simulink model "ComputerPilot"  (R2023b)
settings: Solver=FixedStepAuto  StartTime=0.0  StopTime=inf  FixedStep=sample_time  RelTol=1e-3
InitFcn:
  | load("drone_buses.mat");
model workspace (MAT data in the model file):
  SL_ROS_VariableLengthArrays_MaxSizes.CommonInfo.ArrayTruncateAction = 'EmitWarning'
  SL_ROS_VariableLengthArrays_MaxSizes.MsgTypeMap = containers.Map
  SL_ROS_VariableLengthArrays_MaxSizes.MsgTypeMap.serialization.keys = {'sensor_msgs/Image'}
  SL_ROS_VariableLengthArrays_MaxSizes.MsgTypeMap.serialization.values{1}(1).PropertyName = 'data'
  SL_ROS_VariableLengthArrays_MaxSizes.MsgTypeMap.serialization.values{1}(1).DataType = 'uint8'
  SL_ROS_VariableLengthArrays_MaxSizes.MsgTypeMap.serialization.values{1}(1).MaxLength = 921600
  SL_ROS_VariableLengthArrays_MaxSizes.MsgTypeMap.serialization.values{1}(2).PropertyName = 'encoding'
  SL_ROS_VariableLengthArrays_MaxSizes.MsgTypeMap.serialization.values{1}(2).DataType = 'uint8'
  SL_ROS_VariableLengthArrays_MaxSizes.MsgTypeMap.serialization.values{1}(2).MaxLength = 128
  SL_ROS_VariableLengthArrays_MaxSizes.MsgTypeMap.serialization.uniformity = 0
  SL_ROS_VariableLengthArrays_MaxSizes.MsgTypeMap.serialization.keyType = 'char'
  SL_ROS_VariableLengthArrays_MaxSizes.MsgTypeMap.serialization.valueType = 'any'
  sample_time = 0.1
undefined symbols (not defined in the file): duration, vel
libraries: ros2lib x5, visionsinks x1
settings Model: Creator=rcasado  LastModifiedBy=Rafa
settings SolverCC: AlgebraicLoopSolver=TrustRegion
settings DataIOCC: ReturnWorkspaceOutputs=off
settings OptimizationCC: EnhancedBackFolding=on  PassReuseOutputArgsAs=Individual arguments  ZeroExternalMemoryAtStartup=off  ZeroInternalMemoryAtStartup=off  MaxStackSize=64  OptimizeBlockOrder=speed  DifferentSizesBufferReuse=on  OptimizationCustomize=off  EfficientTunableParamExpr=on
settings DebuggingCC: ParameterTunabilityLossMsg=error  UnconnectedInputMsg=warning  UnconnectedOutputMsg=warning  UnconnectedLineMsg=warning  BusObjectLabelMismatch=none  PregeneratedLibrarySubsystemCodeDiagnostic=none  ArithmeticOperatorsInVariantConditions=warning
settings HardwareCC: ProdBitPerPointer=32  ProdBitPerSizeT=32  ProdBitPerPtrDiffT=32  ProdLargestAtomicFloat=None  ProdIntDivRoundTo=Undefined  ProdEndianess=Unspecified  ProdWordSize=32  ProdHWDeviceType=Generic->Unspecified (assume 32-bit Generic)
settings ModelReferenceCC: EnableRefExpFcnMdlSchedulingChecks=on
settings SFSimCC: SimUseLocalCustomCode=off  CustomCodeUndefinedFunction=UseInterfaceOnly  SimTargetLang=C++
settings RTWCC: Description=Embedded Coder  SystemTargetFile=ert.tlc  HardwareBoard=Robot Operating System (ROS)  TLCOptions="-aInlineSetEventsForThisBaseRateFcn=TLC_FALSE -aSuppressMultiTaskScheduler=TLC_FALSE  -aRateBasedStepFcn=0"  GenCodeOnly=on  TemplateMakefile=ert_default_tmf  GenerateReport=on  RTWUseLocalCustomCode=off  Toolchain=Catkin  IncludeHyperlinkInReport=on  LaunchReport=on  TargetLang=C++  GenerateTraceInfo=on  GenerateTraceReport=on  GenerateTraceReportSl=on  GenerateTraceReportSf=on  GenerateTraceReportEml=on  DLArmComputeVersion=19.05
settings CodeAppCC: ForceParamTrailComments=on  IgnoreCustomStorageClasses=off  OperatorAnnotations=on  SimulinkDataObjDesc=on  SFDataObjDesc=on  InsertBlockDesc=on

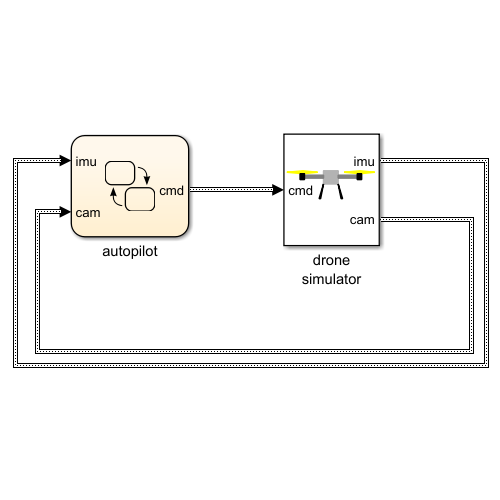
[thumbnail: Simulink's stored preview of the top-level diagram]
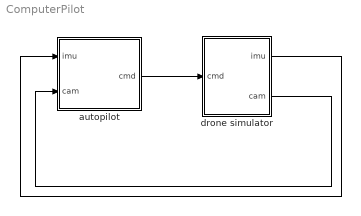
== system ComputerPilot ==
  autopilot : Stateflow chart  TreatAsAtomicUnit=on
  drone simulator : Subsystem
      mask Display:
      | patch([50 -50 -50 50], [40 40 -60 -60], [1 1 1])
      | 
      | patch([8 -8 -8 8], [6 6 -6 -6], [0.7 0.7 0.7])
      | 
      | patch([ 8  8  28  28], [2 0 0 2], [0.5 0.5 0.5])
      | patch([-8 -8 -28 -28], [2 0 0 2], [0.5 0.5 0.5])
      | 
      | patch([ 30  46  30  14], [6 5 4 5], [1 1 0])
      | patch([-30 -46 -30 -14], [6 5 4 5], [1 1 0])
      | 
      | patch([ 28  28  32  32], [4 -2 -2 4], [0 0 0])
      | patch([-28 -28 -32 -32], [4 -2 -2 4], [0 0 0])
      | 
      | patch([ 8  12  11  7], [-6 -18 -18 -6], [0 0 0])
      | patch([-8 -12 -11 -7], [-6 -18 -18 -6], [0 0 0])
  wires:
  drone simulator/1(imu) -> autopilot/1(imu)
  autopilot/1(cmd) -> drone simulator/1(cmd)
  drone simulator/2(cam) -> autopilot/2(cam)

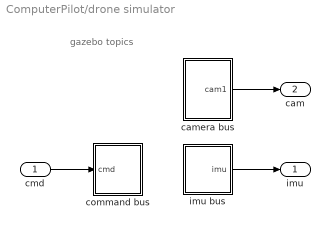
== system ComputerPilot/drone simulator ==
  note: gazebo
      | topics
  cmd : Inport
  camera bus : Subsystem
  command bus : Subsystem
  imu bus : Subsystem
  imu : Outport  VectorParamsAs1DForOutWhenUnconnected=off
  cam : Outport  Port=2  VectorParamsAs1DForOutWhenUnconnected=off
  wires:
  imu bus/1(imu) -> imu/1
  cmd/1 -> command bus/1(cmd)
  camera bus/1(cam1) -> cam/1

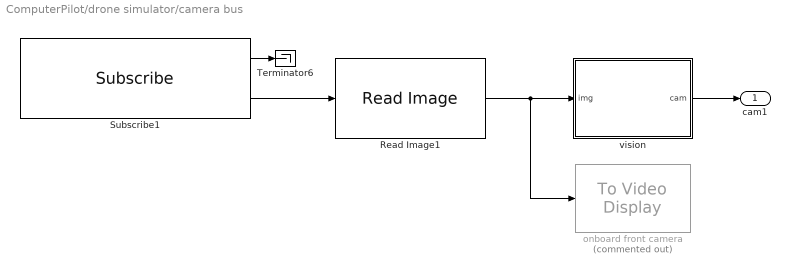
== system ComputerPilot/drone simulator/camera bus ==
  Read Image1 : ros2lib/Read Image  MaximumImageSize=[240, 320]  ImageEncoding=rgb8  ShowAlphaOutput=off  ShowErrorCodeOutput=off  VariableSizeOutputs=off
  Subscribe1 : ros2lib/Subscribe  topicSource=Select from ROS network  topic=/NavSim/abejorro/onboard_cam/image_raw  messageType=sensor_msgs/Image  sampleTime=0.1  QOSHistory=Keep last  QOSDepth=1  QOSReliability=Reliable  QOSDurability=Volatile
  Terminator6 : Terminator
  onboard front camera : visionsinks/To Video Display  Commented=on  windowSizeMode=Normal  openAtMdlStart=on  fullScreen=off  videoWindowX=536805376  videoWindowY=536805376  saveWindowSize=off  videoWindowWidth=479  videoWindowHeight=321  inputColorFormat=RGB  inputType=Obsolete  imagePorts=One multidimensional signal  OutputDevice=On-screen video monitor  dataOrg=Column-major  isWindowOpen=off
  vision : MATLAB Function  TreatAsAtomicUnit=on
  cam1 : Outport  VectorParamsAs1DForOutWhenUnconnected=off
  wires:
  Subscribe1/2 -> Read Image1/1
  vision/1(cam) -> cam1/1
  Subscribe1/1 -> Terminator6/1
  Read Image1/1 -> vision/1(img), onboard front camera/1

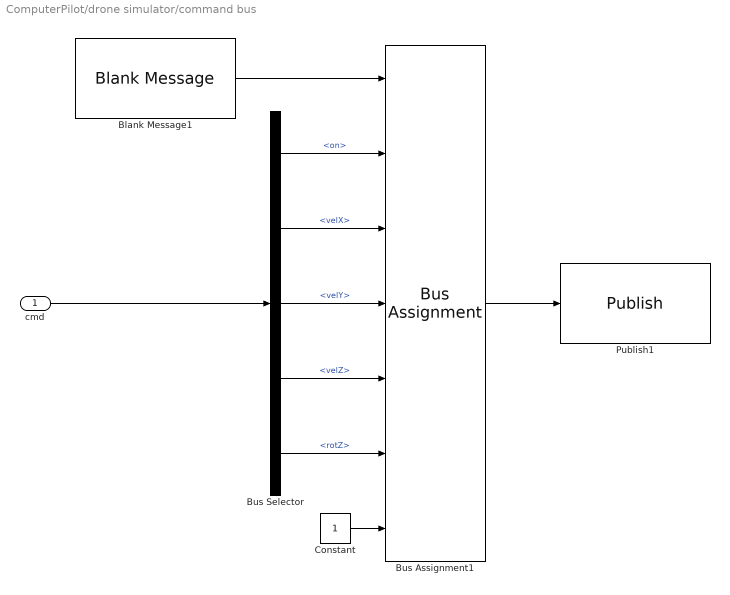
== system ComputerPilot/drone simulator/command bus ==
  cmd : Inport
  Blank Message1 : ros2lib/Blank Message  messageClass=Message  entityType=navsim_msgs/RemoteCommand  messageType=navsim_msgs/RemoteCommand  SampleTime=sample_time
  Bus Assignment1 : BusAssignment  AssignedSignals=on,vel.linear.x,vel.linear.y,vel.linear.z,vel.angular.z,duration.sec
  Bus Selector : BusSelector  OutputSignals=on,velX,velY,velZ,rotZ
  Constant : Constant  OutDataTypeStr=int32
  Publish1 : ros2lib/Publish  topicSource=Select from ROS network  topic=/NavSim/abejorro/RemoteCommand  messageType=navsim_msgs/RemoteCommand  QOSHistory=Keep last  QOSDepth=1  QOSReliability=Reliable  QOSDurability=Volatile
  wires:
  cmd/1 -> Bus Selector/1
  Bus Selector/4 -> Bus Assignment1/5  "<velZ>"
  Bus Selector/3 -> Bus Assignment1/4  "<velY>"
  Bus Selector/2 -> Bus Assignment1/3  "<velX>"
  Bus Selector/1 -> Bus Assignment1/2  "<on>"
  Bus Selector/5 -> Bus Assignment1/6  "<rotZ>"
  Blank Message1/1 -> Bus Assignment1/1
  Bus Assignment1/1 -> Publish1/1
  Constant/1 -> Bus Assignment1/7

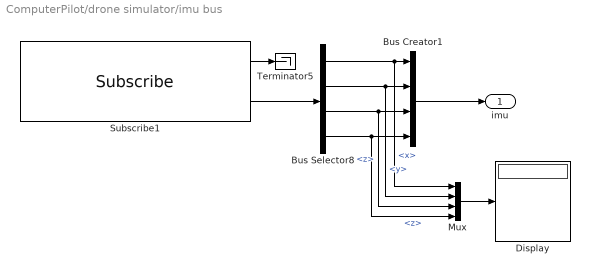
== system ComputerPilot/drone simulator/imu bus ==
  Bus Creator1 : BusCreator  Inputs=4  OutDataTypeStr=Bus: bus_IMU  NonVirtualBus=on
      settings: InheritFromInputs=off
  Bus Selector8 : BusSelector  DialogController=Simulink.DDGSource_BusSelector  OutputSignals=pose.position.x,pose.position.y,pose.position.z,pose.orientation.z
  Display : Display
  Mux : Mux
  Subscribe1 : ros2lib/Subscribe  topicSource=Select from ROS network  topic=/NavSim/abejorro/Telemetry  messageType=navsim_msgs/Telemetry  sampleTime=0.1  QOSHistory=Keep last  QOSDepth=1  QOSReliability=Reliable  QOSDurability=Volatile
  Terminator5 : Terminator
  imu : Outport  VectorParamsAs1DForOutWhenUnconnected=off
  wires:
  Subscribe1/1 -> Terminator5/1
  Bus Selector8/4 -> Mux/4, Bus Creator1/4  "<z>"
  Bus Selector8/1 -> Mux/1, Bus Creator1/1  "<x>"
  Bus Creator1/1 -> imu/1
  Subscribe1/2 -> Bus Selector8/1
  Bus Selector8/2 -> Mux/2, Bus Creator1/2  "<y>"
  Bus Selector8/3 -> Mux/3, Bus Creator1/3  "<z>"
  Mux/1 -> Display/1

== stateflow chart ComputerPilot/autopilot ==
  settings: updateMethod=DISCRETE  sampleTime=sample_time  executeAtInitialization=1
  state RedFrame
    state Go2Center
      entry:
    state FrameVisible
      entry:
      Hover();
      during:
      Look2Frame('red');
      cmd.velX = min((cam.red.d-0.4)/2,0.2);
    state Turning
      entry:
      Hover();
      cmd.rotZ = 0.5;
    state FrameClose
      entry:
      Hover
      initA = cam.red.a
    state ShiftLeft
      entry:
      cmd.velY = 0.05;
      during:
      Look2Frame('red');
      cmd.velX = (cam.red.d-0.3)/10;
    state ShiftRight
      entry:
      cmd.velY = -0.01;
      during:
      Look2Frame('red');
      cmd.velX = (cam.red.d-0.3)/10;
    state Crossing
      entry:
      Hover
      cmd.velX = 0.1;
      during:
      Look2Frame('red');
    state GoingUp
      entry:
      Hover
      cmd.velZ = 0.2;
    state End
    (default) -> RedFrame.Go2Center
    RedFrame.Go2Center -> RedFrame.FrameVisible [order 1] : [cam.red.d ~= inf]
    RedFrame.FrameVisible -> RedFrame.Go2Center [order 2] : [cam.red.d == inf]
    RedFrame.Go2Center -> RedFrame.Turning [order 2] : [Fly2(0, 0, 1)<0.2]
    RedFrame.Turning -> RedFrame.FrameVisible : [cam.red.d ~= inf]
    RedFrame.FrameVisible -> RedFrame.FrameClose [order 1] : [cam.red.d < 0.5]
    RedFrame.FrameClose -> RedFrame.ShiftLeft
    RedFrame.ShiftLeft -> RedFrame.ShiftRight [order 2] : [initA < cam.red.a]
    RedFrame.ShiftRight -> RedFrame.Crossing : [cam.red.a < 3]
    RedFrame.ShiftLeft -> RedFrame.Crossing [order 1] : [cam.red.a < 3]
    RedFrame.Crossing -> RedFrame.GoingUp : [after(10,sec)]
    RedFrame.GoingUp -> RedFrame.End : [after(4,sec)]
  state GreenFrame
    state Go2Center
      entry:
    state FrameVisible
      entry:
      Hover();
      during:
      Look2Frame('green');
      cmd.velX = min((cam.green.d-0.4)/2,0.2);
    state Turning
      entry:
      Hover();
      cmd.rotZ = 0.5;
    state FrameClose
      entry:
      Hover
      initA = cam.green.a
    state ShiftLeft
      entry:
      cmd.velY = 0.1;
      during:
      Look2Frame('green');
      cmd.velX = (cam.green.d-0.3)/10;
    state ShiftRight
      entry:
      cmd.velY = -0.1;
      during:
      Look2Frame('green');
      cmd.velX = (cam.green.d-0.3)/10;
    state Crossing
      entry:
      Hover
      cmd.velX = 0.1;
      during:
      Look2Frame('green');
    state GoingUp
      entry:
      Hover
      cmd.velZ = 0.2;
    state End
    (default) -> GreenFrame.Go2Center
    GreenFrame.Go2Center -> GreenFrame.FrameVisible [order 1] : [cam.green.d ~= inf]
    GreenFrame.FrameVisible -> GreenFrame.Go2Center [order 2] : [cam.green.d == inf]
    GreenFrame.Go2Center -> GreenFrame.Turning [order 2] : [Fly2(0, 0, 1)<0.2]
    GreenFrame.Turning -> GreenFrame.FrameVisible : [cam.green.d ~= inf]
    GreenFrame.FrameVisible -> GreenFrame.FrameClose [order 1] : [cam.green.d < 0.5]
    GreenFrame.FrameClose -> GreenFrame.ShiftLeft
    GreenFrame.ShiftLeft -> GreenFrame.ShiftRight [order 2] : [initA < cam.green.a]
    GreenFrame.ShiftRight -> GreenFrame.Crossing : [cam.green.a < 3]
    GreenFrame.ShiftLeft -> GreenFrame.Crossing [order 1] : [cam.green.a < 3]
    GreenFrame.Crossing -> GreenFrame.GoingUp : [after(10,sec)]
    GreenFrame.GoingUp -> GreenFrame.End : [after(4,sec)]
  state BlueFrame
    state Go2Center
      entry:
    state FrameVisible
      entry:
      Hover();
      during:
      Look2Frame('blue');
      cmd.velX = min((cam.blue.d-0.4)/2,0.2);
    state Turning
      entry:
      Hover();
      cmd.rotZ = 0.5;
    state FrameClose
      entry:
      Hover
      initA = cam.blue.a
    state ShiftLeft
      entry:
      cmd.velY = 0.05;
      during:
      Look2Frame('blue');
      cmd.velX = (cam.blue.d-0.3)/10;
    state ShiftRight
      entry:
      cmd.velY = -0.1;
      during:
      Look2Frame('blue');
      cmd.velX = (cam.blue.d-0.3)/10;
    state Crossing
      entry:
      Hover
      cmd.velX = 0.1;
      during:
      Look2Frame('blue');
    state GoingUp
      entry:
      Hover
      cmd.velZ = 0.2;
    state End
    (default) -> BlueFrame.Go2Center
    BlueFrame.Go2Center -> BlueFrame.FrameVisible [order 1] : [cam.blue.d ~= inf]
    BlueFrame.FrameVisible -> BlueFrame.Go2Center [order 2] : [cam.blue.d == inf]
    BlueFrame.Go2Center -> BlueFrame.Turning [order 2] : [Fly2(0, 0, 1)<0.2]
    BlueFrame.Turning -> BlueFrame.FrameVisible : [cam.blue.d ~= inf]
    BlueFrame.FrameVisible -> BlueFrame.FrameClose [order 1] : [cam.blue.d < 0.5]
    BlueFrame.FrameClose -> BlueFrame.ShiftLeft
    BlueFrame.ShiftLeft -> BlueFrame.ShiftRight [order 2] : [initA < cam.blue.a]
    BlueFrame.ShiftRight -> BlueFrame.Crossing : [cam.blue.a < 3]
    BlueFrame.ShiftLeft -> BlueFrame.Crossing [order 1] : [cam.blue.a < 3]
    BlueFrame.Crossing -> BlueFrame.GoingUp : [after(10,sec)]
    BlueFrame.GoingUp -> BlueFrame.End : [after(4,sec)]
  state TakeOff
    state End
    state SetBase
      entry:
      posXinit = imu.posX;
      posYinit = imu.posY;
      posZinit = imu.posZ;
    state Start
      entry:
      Hover();
    SetBase -> TakeOff.End : [Fly2(posXinit, posYinit, 1)<0.1]
    Start -> SetBase : after(1,sec)
    (default) -> Start
  state Landing
    state Go2Base
    state Stop
      entry:
      cmd.on = false;
    (default) -> Go2Base
    Go2Base -> Stop : [Fly2(posXinit, posYinit, 0.6)<0.05]
  TakeOff.End -> RedFrame
  (default) -> TakeOff
  RedFrame.End -> GreenFrame
  GreenFrame.End -> BlueFrame
  BlueFrame.End -> Landing
  data: X function_input; d3D function_output; Y function_input; Z function_input; id function_input; imu input Bus: bus_IMU size=1; cmd output Bus: bus_command size=1 =0; cam input Bus: bus_camera size=1; posZinit local; posYinit local; posXinit local; initA local
  function d3D = Fly2(X,Y,Z):
    | function d3D = Fly2(X,Y,Z)
    | 
    | % target distance decomposed into earth axes
    | dxe = X - imu.posX;
    | dye = Y - imu.posY;
    | dze = Z - imu.posZ;
    | 
    | % target distance
    | d3D = norm([dxe;dye;dze]);
    | 
    | % target distance on the plane
    | d2D = norm([dxe;dye]);
    | 
    | % angle between drone heading and target
    | bearing = rad2deg(atan2(dye, dxe) - imu.rumbo);
    | 
    | % target distance decomposed into drone body axes
    | dx = d2D * cosd(bearing);
    | dy = d2D * sind(bearing);
    | dz = dze;
    | 
    | % velocity obtained from distance
    | vel = [dx;dy;dz]/2;
    | if norm(vel) > 0.2 
    |     vel = vel / norm(vel);
    |     vel = vel * 0.2;
    | end
    | 
    | cmd.velX = vel(1);
    | cmd.velY = vel(2);
    | cmd.velZ = vel(3);
  function Hover:
    | function Hover
    | 
    | cmd.on   = true;
    | cmd.velX = 0;
    | cmd.velY = 0;
    | cmd.velZ = 0;
    | cmd.rotZ = 0;
  function Look2Frame(id):
    | function Look2Frame(id)
    | 
    | switch id
    |     case 'red'
    |         fr = cam.red;
    |     case 'green'
    |         fr = cam.green;
    |     case 'blue'
    |         fr = cam.blue;
    | end
    | 
    | if (fr.d ~= inf)
    |     HorCenter = (fr.e + fr.w)/2;
    |     cmd.rotZ  = - HorCenter/250;
    |     VerCenter = (fr.n + fr.s)/2;
    |     cmd.velZ  = VerCenter/400;
    | end

== matlab function ComputerPilot/drone simulator/camera bus/vision ==
  data: img input; cam output Bus: bus_camera
function cam = fcn(img)

% Procesamos la imagen, que debe ser de 320x240 pixeles
% figName = 'pilot camera';
% figHandler = findobj('Type','figure','Name',figName)';
% 
% if isempty(figHandler) 
%     % la figura no existe, hay que construirla
%     figHandler = figure( ...
%         'Name',figName, ...
%         'NumberTitle','off', ...
%         'MenuBar', 'none', ...
%         'Resize','on');
% 
%     % eje dentro de la figura
%     axesHandler = axes(      ...
%       'Parent', figHandler,  ...
%       'Units','normalized', ...
%       'Visible','on');
%     grid(axesHandler,'on');
%     hold(axesHandler,'on');
%     axis equal
%     axis([-160 160 -120 120])
% 
% end
% 
% coder.extrinsic('imshow');
% imshow(img);
% 







% establecemos los valores umbrales de deteccion de color
th1 = 50;         % umbral entre color primario y secundarios
th2 = 20;         % umbral entre colores secundarios

% marco rojo
frame_red.d = +inf;        % distancia estimada
frame_red.a = +inf;        % angulo de entrada estimado
frame_red.n = +inf;        % lado norte
frame_red.s = -inf;        % lado sur
frame_red.e = -inf;        % lado este
frame_red.w = +inf;        % lado oeste

% marco verde
frame_green = frame_red;      
% marco azul
frame_blue = frame_red; 


% deteccion de rectangulos conteniendo los pixeles de cada marco
for row = 1:240
for col = 1:320

    r = double(img(row,col,1));
    g = double(img(row,col,2));
    b = double(img(row,col,3)); 

    if(abs(g-b) < th2) && ((r-g) > th1)        %rojo
        if(frame_red.n > row) 
           frame_red.n = double(row);
        end
        if(frame_red.s < row) 
           frame_red.s = double(row);
        end
        if(frame_red.e < col) 
           frame_red.e = double(col);
        end
        if(frame_red.w > col) 
           frame_red.w = double(col);
        end
    elseif(abs(b-r) < th2) && ((g-b) > th1)    %verde
        if(frame_green.n > row) 
           frame_green.n = double(row);
        end
        if(frame_green.s < row) 
           frame_green.s = double(row);
        end
        if(frame_green.e < col) 
           frame_green.e = double(col);
        end
        if(frame_green.w > col) 
           frame_green.w = double(col);
        end
    elseif(abs(r-g) < th2) && ((b-r) > th1)    %azul
        if(frame_blue.n > row) 
           frame_blue.n = double(row);
        end
        if(frame_blue.s < row) 
           frame_blue.s = double(row);
        end
        if(frame_blue.e < col) 
           frame_blue.e = double(col);
        end
        if(frame_blue.w > col) 
           frame_blue.w = double(col);
        end
    end

end
end

% Cambio del sistema de coordenadas de la imagen
frame_red.n   = 120 - frame_red.n;
frame_red.s   = 120 - frame_red.s;
frame_red.e   = frame_red.e - 161;
frame_red.w   = frame_red.w - 161;

frame_green.n = 120 - frame_green.n;
frame_green.s = 120 - frame_green.s;
frame_green.e = frame_green.e - 161;
frame_green.w = frame_green.w - 161;

frame_blue.n  = 120 - frame_blue.n;
frame_blue.s  = 120 - frame_blue.s;
frame_blue.e  = frame_blue.e - 161;
frame_blue.w  = frame_blue.w - 161;


%% Analisis de posicion (distancia, y angulos de deriva/entrada)

d2 = 160^2;    % 160^2 pixeles
L  = 0.23;       % alto de marco
A  = 0.43;       % ancho del marco

if frame_red.n > -inf && frame_red.n < 119 && frame_red.s > -120
    l = frame_red.n - frame_red.s;
    h = frame_red.s + l/2;
    frame_red.d = L/l * sqrt(d2 + h^2);
    ap = frame_red.e - frame_red.w;
    a = max(A/L * l,ap);
    frame_red.a = acosd(ap/a);
end

if frame_green.n > -inf && frame_green.n < 119 && frame_green.s > -120
    l = frame_green.n - frame_green.s;
    h = frame_green.s + l/2;
    frame_green.d = L/l * sqrt(d2 + h^2);
    ap = frame_green.e - frame_green.w;
    a = max(A/L * l,ap);
    frame_green.a = acosd(ap/a);
end

if frame_blue.n > -inf && frame_blue.n < 119 && frame_blue.s > -120
    l = frame_blue.n - frame_blue.s;
    h = frame_blue.s + l/2;
    frame_blue.d = L/l * sqrt(d2 + h^2);
    ap = frame_blue.e - frame_blue.w;
    a = max(A/L * l,ap);
    frame_blue.a = acosd(ap/a);
end




%% Enviamos informacion por el topic
cam.red = frame_red;
cam.green = frame_green;
cam.blue = frame_blue;
